simulink model "sys1sys2solucheck"  (R2018b)
settings: Solver=ode45  StartTime=0.0  StopTime=100  RelTol=1e-3  EnableMultiTasking=on
settings Model: Creator=wzhan174  LastModifiedBy=Jacob
settings DataIOCC: LimitDataPoints=on  SaveFormat=Array
settings OptimizationCC: LifeSpan=inf
settings DebuggingCC: SFUnexpectedBacktrackingDiag=warning  SFNoUnconditionalDefaultTransitionDiag=warning  SFExecutionAtInitializationDiag=none
settings HardwareCC: ProdBitPerPointer=32  ProdBitPerSizeT=32  ProdBitPerPtrDiffT=32  ProdLargestAtomicFloat=None  ProdIntDivRoundTo=Undefined  ProdEndianess=Unspecified  ProdWordSize=32  ProdHWDeviceType=32-bit Generic
settings ModelReferenceCC: PropagateSignalLabelsOutOfModel=off
settings SFSimCC: SimUseLocalCustomCode=off
settings RTWCC: RTWUseLocalCustomCode=off
settings CodeAppCC: StateflowObjectComments=on
settings GRTTargetCC: TargetLangStandard=C89/C90 (ANSI)  GeneratePreprocessorConditionals=Disable all
settings ConfigComp: CovMetricSettings=dw  CovHtmlReporting=on  CovSaveCumulativeToWorkspaceVar=on  CovSaveSingleToWorkspaceVar=on  CovExternalEMLEnable=off

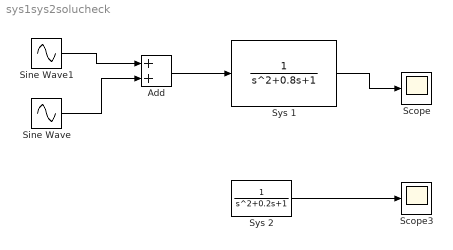
== system sys1sys2solucheck ==
  Add : Sum
  Scope : Scope
  Scope3 : Scope
  Sine Wave : Sin  Amplitude=6  Frequency=0.1  SampleTime=0
  Sine Wave1 : Sin  Amplitude=0.5  SampleTime=0
  Sys 1 : TransferFcn  Denominator=[1 0.8 1]
  Sys 2 : TransferFcn  Denominator=[1 0.2 1]
  wires:
  Sys 1/1 -> Scope/1
  Sys 2/1 -> Scope3/1
  Add/1 -> Sys 1/1
  Sine Wave1/1 -> Add/1
  Sine Wave/1 -> Add/2
